simulink model "gm_Phase_voltages_per_switching_state_MPC_6Phase"  (R2022a)
settings: Solver=FixedStepDiscrete  StartTime=0.0  StopTime=10.0  RelTol=1e-3
undefined symbols (not defined in the file or in its folder): f_c, u_dc
libraries: hdlmdlgenlib x9
settings Model: Creator=Andre Merx  LastModifiedBy=Andre Merx
settings SolverCC: AlgebraicLoopSolver=TrustRegion
settings DataIOCC: LimitDataPoints=on  SaveOutput=off  SaveTime=off
settings OptimizationCC: BlockReduction=off  ConditionallyExecuteInputs=off  DefaultParameterBehavior=Inlined  LifeSpan=inf
settings DebuggingCC: AlgebraicLoopMsg=error  InheritedTsInSrcMsg=none  SingleTaskRateTransMsg=error  UnconnectedInputMsg=warning  UnconnectedOutputMsg=warning  UnconnectedLineMsg=warning  AllowSymbolicDim=off  StrictBusMsg=ErrorOnBusTreatedAsVector  SFUnexpectedBacktrackingDiag=warning  SFNoUnconditionalDefaultTransitionDiag=warning  SFExecutionAtInitializationDiag=none  SFMachineParentedDataDiag=warning  ArithmeticOperatorsInVariantConditions=warning
settings HardwareCC: ProdBitPerPointer=32  ProdBitPerSizeT=32  ProdBitPerPtrDiffT=32  ProdLargestAtomicFloat=None  ProdIntDivRoundTo=Undefined  ProdEndianess=Unspecified  ProdWordSize=32  ProdHWDeviceType=ASIC/FPGA->ASIC/FPGA  ProdEqTarget=off
settings SFSimCC: SimUseLocalCustomCode=off  CustomCodeUndefinedFunction=UseInterfaceOnly
settings RTWCC: RTWUseLocalCustomCode=off
settings CodeAppCC: StateflowObjectComments=on
settings GRTTargetCC: TargetLangStandard=C89/C90 (ANSI)
settings ConfigComp: CovScope=ReferencedModels  CovMetricSettings=dw  CovSaveCumulativeToWorkspaceVar=on  CovSaveSingleToWorkspaceVar=on  CovExternalEMLEnable=off  CovSFcnEnable=off

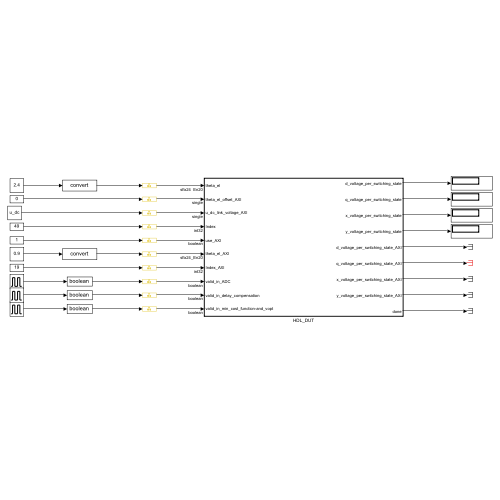
[thumbnail: Simulink's stored preview of the top-level diagram]
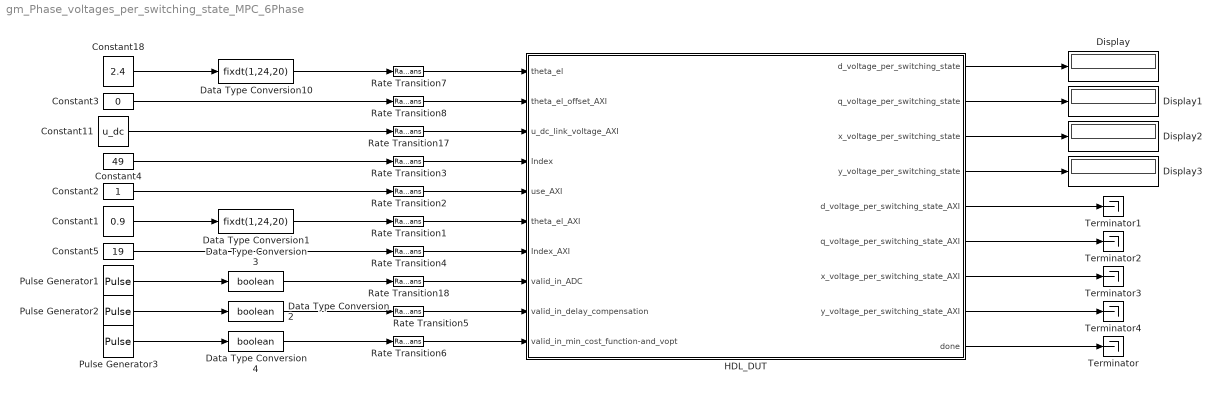
== system gm_Phase_voltages_per_switching_state_MPC_6Phase ==
  Constant1 : Constant  Value=0.9
  Constant11 : Constant  Value=u_dc  OutDataTypeStr=single  SampleTime=-1
  Constant18 : Constant  Value=2.4
  Constant2 : Constant  OutDataTypeStr=boolean  SampleTime=-1
  Constant3 : Constant  Value=0  OutDataTypeStr=single  SampleTime=-1
  Constant4 : Constant  Value=49  OutDataTypeStr=int32  SampleTime=-1
  Constant5 : Constant  Value=19  OutDataTypeStr=int32  SampleTime=-1
  Data Type Conversion1 : DataTypeConversion  OutDataTypeStr=fixdt(1,24,20)  SaturateOnIntegerOverflow=off  RndMeth=Floor
  Data Type Conversion10 : DataTypeConversion  OutDataTypeStr=fixdt(1,24,20)  SaturateOnIntegerOverflow=off  RndMeth=Floor
  Data Type Conversion2 : DataTypeConversion  OutDataTypeStr=boolean  SaturateOnIntegerOverflow=off  RndMeth=Floor
  Data Type Conversion3 : DataTypeConversion  OutDataTypeStr=boolean  SaturateOnIntegerOverflow=off  RndMeth=Floor
  Data Type Conversion4 : DataTypeConversion  OutDataTypeStr=boolean  SaturateOnIntegerOverflow=off  RndMeth=Floor
  Display{,1..3} (4 alike) : Display
  HDL_DUT : Subsystem  TreatAsAtomicUnit=on
  Pulse Generator1 : DiscretePulseGenerator  PulseType=Time based  Period=1/f_c
  Pulse Generator2 : DiscretePulseGenerator  PulseType=Time based  Period=1/f_c
  Pulse Generator3 : DiscretePulseGenerator  PulseType=Time based  Period=1/f_c
  Rate Transition{1..8,17..18} (10 alike) : RateTransition  OutPortSampleTime=Rt
  Terminator{,1..4} (5 alike) : Terminator
  wires:
  HDL_DUT/9(done) -> Terminator/1
  Rate Transition6/1 -> HDL_DUT/10(valid_in_min_cost_function-and_vopt)
  Data Type Conversion4/1 -> Rate Transition6/1
  Pulse Generator3/1 -> Data Type Conversion4/1
  Rate Transition5/1 -> HDL_DUT/9(valid_in_delay_compensation)
  Data Type Conversion2/1 -> Rate Transition5/1
  Pulse Generator2/1 -> Data Type Conversion2/1
  HDL_DUT/8(y_voltage_per_switching_state_AXI) -> Terminator4/1
  HDL_DUT/7(x_voltage_per_switching_state_AXI) -> Terminator3/1
  HDL_DUT/6(q_voltage_per_switching_state_AXI) -> Terminator2/1
  HDL_DUT/5(d_voltage_per_switching_state_AXI) -> Terminator1/1
  Rate Transition4/1 -> HDL_DUT/7(Index_AXI)
  Constant5/1 -> Rate Transition4/1
  Rate Transition3/1 -> HDL_DUT/4(Index)
  Constant4/1 -> Rate Transition3/1
  HDL_DUT/4(y_voltage_per_switching_state) -> Display3/1
  HDL_DUT/3(x_voltage_per_switching_state) -> Display2/1
  HDL_DUT/2(q_voltage_per_switching_state) -> Display1/1
  HDL_DUT/1(d_voltage_per_switching_state) -> Display/1
  Rate Transition2/1 -> HDL_DUT/5(use_AXI)
  Constant2/1 -> Rate Transition2/1
  Rate Transition1/1 -> HDL_DUT/6(theta_el_AXI)
  Constant1/1 -> Data Type Conversion1/1
  Data Type Conversion1/1 -> Rate Transition1/1
  Rate Transition18/1 -> HDL_DUT/8(valid_in_ADC)
  Data Type Conversion3/1 -> Rate Transition18/1
  Pulse Generator1/1 -> Data Type Conversion3/1
  Rate Transition8/1 -> HDL_DUT/2(theta_el_offset_AXI)
  Constant18/1 -> Data Type Conversion10/1
  Constant3/1 -> Rate Transition8/1
  Rate Transition7/1 -> HDL_DUT/1(theta_el)
  Rate Transition17/1 -> HDL_DUT/3(u_dc_link_voltage_AXI)
  Data Type Conversion10/1 -> Rate Transition7/1
  Constant11/1 -> Rate Transition17/1

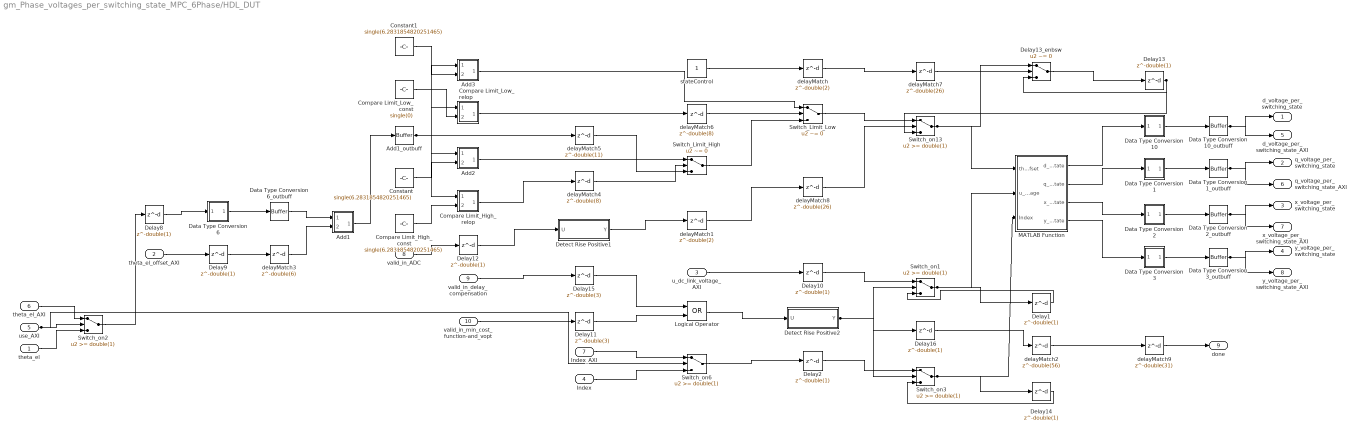
== system gm_Phase_voltages_per_switching_state_MPC_6Phase/HDL_DUT ==
  theta_el : Inport  OutDataTypeStr=fixdt(1, 24, 20)  PortDimensions=1  SampleTime=1e-08
  theta_el_offset_AXI : Inport  Port=2  OutDataTypeStr=single  PortDimensions=1  SampleTime=1e-08
  u_dc_link_voltage_AXI : Inport  Port=3  OutDataTypeStr=single  PortDimensions=1  SampleTime=1e-08
  Index : Inport  Port=4  OutDataTypeStr=int32  PortDimensions=1  SampleTime=1e-08
  use_AXI : Inport  Port=5  OutDataTypeStr=boolean  PortDimensions=1  SampleTime=1e-08
  theta_el_AXI : Inport  Port=6  OutDataTypeStr=fixdt(1, 24, 20)  PortDimensions=1  SampleTime=1e-08
  Index_AXI : Inport  Port=7  OutDataTypeStr=int32  PortDimensions=1  SampleTime=1e-08
  valid_in_ADC : Inport  Port=8  OutDataTypeStr=boolean  PortDimensions=1  SampleTime=1e-08
  valid_in_delay_compensation : Inport  Port=9  OutDataTypeStr=boolean  PortDimensions=1  SampleTime=1e-08
  valid_in_min_cost_function-and_vopt : Inport  Port=10  OutDataTypeStr=boolean  PortDimensions=1  SampleTime=1e-08
  Add1 : Subsystem
      mask Display: disp('NFP\nadd');
  Add1_outbuff : hdlmdlgenlib/Buffer
      settings: SourceProductBaseCode=SL
  Add2 : Subsystem
      mask Display: disp('NFP\nadd');
  Add3 : Subsystem
      mask Display: disp('NFP\nadd');
  Compare Limit_High_const : Constant  Value=single(6.2831854820251465)  OutDataTypeStr=single  SampleTime=1e-08
  Compare Limit_High_relop : Subsystem
      mask Display: disp('NFP\nrelop');
  Compare Limit_Low_const : Constant  Value=single(0)  OutDataTypeStr=single  SampleTime=1e-08
  Compare Limit_Low_relop : Subsystem
      mask Display: disp('NFP\nrelop');
  Constant : Constant  Value=single(6.2831854820251465)  OutDataTypeStr=single  SampleTime=1e-08
  Constant1 : Constant  Value=single(6.2831854820251465)  OutDataTypeStr=single  SampleTime=1e-08
  Data Type Conversion1 : Subsystem
      mask Display: disp('NFP\nconv');
  Data Type Conversion10 : Subsystem
      mask Display: disp('NFP\nconv');
  Data Type Conversion10_outbuff : hdlmdlgenlib/Buffer
      settings: SourceProductBaseCode=SL
  Data Type Conversion1_outbuff : hdlmdlgenlib/Buffer
      settings: SourceProductBaseCode=SL
  Data Type Conversion2 : Subsystem
      mask Display: disp('NFP\nconv');
  Data Type Conversion2_outbuff : hdlmdlgenlib/Buffer
      settings: SourceProductBaseCode=SL
  Data Type Conversion3 : Subsystem
      mask Display: disp('NFP\nconv');
  Data Type Conversion3_outbuff : hdlmdlgenlib/Buffer
      settings: SourceProductBaseCode=SL
  Data Type Conversion6 : Subsystem
      mask Display: disp('NFP\nconv');
  Data Type Conversion6_outbuff : hdlmdlgenlib/Buffer
      settings: SourceProductBaseCode=SL
  Delay{1..2,8..10,12..14,16} (9 alike) : Delay  DelayLength=double(1)  InitialCondition=0  SampleTime=1e-08
  Delay11 : Delay  DelayLength=double(3)  InitialCondition=0  SampleTime=1e-08
  Delay13_enbsw : Switch  Criteria=u2 ~= 0  Threshold=double(0)  OutDataTypeStr=single  SampleTime=1e-08  SaturateOnIntegerOverflow=off  InputSameDT=off
  Delay15 : Delay  DelayLength=double(3)  InitialCondition=0  SampleTime=1e-08
  Detect Rise Positive1 : Subsystem  mask(Detect Rise Positive){vinit=double(0), InputProcessing=Elements as channels (sample based), OutDataTypeStr=boolean}
      mask prompts: vinit "Simulink:masks:InitialCondition_MP"; InputProcessing "Simulink:masks:InputProcessing_MP"; OutDataTypeStr "Simulink:masks:OutputDataType_MP"
      mask help: Simulink:masks:DetectRisePositive_MD
      mask init:
      | InputProcessing = 'Elements as channels (sample based)';
      | OutDataTypeStr = 'boolean';
      | vinit = double(0);
      mask TypeOptions InputProcessing: Simulink:masks:ColumnsAsChannelsFrameBased | Simulink:masks:ElementsAsChannelsSampleBased
      mask TypeOptions OutDataTypeStr: Simulink:masks:uint8 | Simulink:masks:boolean
      mask Display: fprintf('U > 0\n&  NOT\nU/z > 0')
  Detect Rise Positive2 : Subsystem  mask(Detect Rise Positive){vinit=double(0), InputProcessing=Elements as channels (sample based), OutDataTypeStr=boolean}
      mask prompts: vinit "Simulink:masks:InitialCondition_MP"; InputProcessing "Simulink:masks:InputProcessing_MP"; OutDataTypeStr "Simulink:masks:OutputDataType_MP"
      mask help: Simulink:masks:DetectRisePositive_MD
      mask init:
      | InputProcessing = 'Elements as channels (sample based)';
      | OutDataTypeStr = 'boolean';
      | vinit = double(0);
      mask TypeOptions InputProcessing: Simulink:masks:ColumnsAsChannelsFrameBased | Simulink:masks:ElementsAsChannelsSampleBased
      mask TypeOptions OutDataTypeStr: Simulink:masks:uint8 | Simulink:masks:boolean
      mask Display: fprintf('U > 0\n&  NOT\nU/z > 0')
  Logical Operator : Logic  Operator=OR  AllPortsSameDT=off  OutDataTypeStr=boolean  SampleTime=1e-08
  MATLAB Function : Subsystem
  Switch_Limit_High : Switch  Criteria=u2 ~= 0  Threshold=double(0)  OutDataTypeStr=single  SampleTime=1e-08  SaturateOnIntegerOverflow=off  InputSameDT=off
  Switch_Limit_Low : Switch  Criteria=u2 ~= 0  Threshold=double(0)  OutDataTypeStr=single  SampleTime=1e-08  SaturateOnIntegerOverflow=off  InputSameDT=off
  Switch_on1 : Switch  Threshold=double(1)  OutDataTypeStr=single  RndMeth=Simplest  SampleTime=1e-08  SaturateOnIntegerOverflow=off  InputSameDT=off
  Switch_on13 : Switch  Threshold=double(1)  OutDataTypeStr=single  RndMeth=Simplest  SampleTime=1e-08  SaturateOnIntegerOverflow=off  InputSameDT=off
  Switch_on2 : Switch  Threshold=double(1)  OutDataTypeStr=fixdt(1, 24, 20)  RndMeth=Simplest  SampleTime=1e-08  SaturateOnIntegerOverflow=off  InputSameDT=off
  Switch_on3 : Switch  Threshold=double(1)  OutDataTypeStr=int32  RndMeth=Simplest  SampleTime=1e-08  SaturateOnIntegerOverflow=off  InputSameDT=off
  Switch_on6 : Switch  Threshold=double(1)  OutDataTypeStr=int32  RndMeth=Simplest  SampleTime=1e-08  SaturateOnIntegerOverflow=off  InputSameDT=off
  delayMatch : Delay  DelayLength=double(2)  InitialCondition=0  SampleTime=1e-08
  delayMatch1 : Delay  DelayLength=double(2)  InitialCondition=0  SampleTime=1e-08
  delayMatch2 : Delay  DelayLength=double(56)  InitialCondition=0  SampleTime=1e-08
  delayMatch3 : Delay  DelayLength=double(6)  InitialCondition=0  SampleTime=1e-08
  delayMatch4 : Delay  DelayLength=double(8)  InitialCondition=0  SampleTime=1e-08
  delayMatch5 : Delay  DelayLength=double(11)  InitialCondition=0  SampleTime=1e-08
  delayMatch6 : Delay  DelayLength=double(8)  InitialCondition=0  SampleTime=1e-08
  delayMatch7 : Delay  DelayLength=double(26)  InitialCondition=0  SampleTime=1e-08
  delayMatch8 : Delay  DelayLength=double(26)  InitialCondition=0  SampleTime=1e-08
  delayMatch9 : Delay  DelayLength=double(31)  InitialCondition=0  SampleTime=1e-08
  stateControl : Constant  OutDataTypeStr=boolean  SampleTime=1e-08
  d_voltage_per_switching_state : Outport  SampleTime=1e-08
  q_voltage_per_switching_state : Outport  Port=2  SampleTime=1e-08
  x_voltage_per_switching_state : Outport  Port=3  SampleTime=1e-08
  y_voltage_per_switching_state : Outport  Port=4  SampleTime=1e-08
  d_voltage_per_switching_state_AXI : Outport  Port=5  SampleTime=1e-08
  q_voltage_per_switching_state_AXI : Outport  Port=6  SampleTime=1e-08
  x_voltage_per_switching_state_AXI : Outport  Port=7  SampleTime=1e-08
  y_voltage_per_switching_state_AXI : Outport  Port=8  SampleTime=1e-08
  done : Outport  Port=9  SampleTime=1e-08
  wires:
  theta_el/1 -> Switch_on2/3
  theta_el_offset_AXI/1 -> Delay9/1
  u_dc_link_voltage_AXI/1 -> Delay10/1
  Index/1 -> Switch_on6/3
  use_AXI/1 -> Switch_on6/2, Switch_on2/2
  theta_el_AXI/1 -> Switch_on2/1
  Index_AXI/1 -> Switch_on6/1
  valid_in_ADC/1 -> Delay12/1
  valid_in_delay_compensation/1 -> Delay15/1
  valid_in_min_cost_function-and_vopt/1 -> Delay11/1
  delayMatch5/1 -> Switch_Limit_High/3
  Constant/1 -> Add2/2(In2)
  Constant1/1 -> Add3/2(In2)
  Data Type Conversion1_outbuff/1 -> q_voltage_per_switching_state/1, q_voltage_per_switching_state_AXI/1
  Data Type Conversion10_outbuff/1 -> d_voltage_per_switching_state_AXI/1, d_voltage_per_switching_state/1
  Data Type Conversion2_outbuff/1 -> x_voltage_per_switching_state_AXI/1, x_voltage_per_switching_state/1
  Data Type Conversion3_outbuff/1 -> y_voltage_per_switching_state/1, y_voltage_per_switching_state_AXI/1
  Data Type Conversion6_outbuff/1 -> Add1/1(In1)
  Delay10/1 -> Switch_on1/1
  Delay11/1 -> Logical Operator/2
  Delay12/1 -> Detect Rise Positive1/1(U)
  Delay15/1 -> Logical Operator/1
  delayMatch9/1 -> done/1
  Delay2/1 -> Switch_on3/1
  Delay8/1 -> Data Type Conversion6/1(In1)
  delayMatch3/1 -> Add1/2(In2)
  delayMatch8/1 -> Switch_on13/2
  Detect Rise Positive2/1(Y) -> Delay16/1, Switch_on1/2, Switch_on3/2
  Logical Operator/1 -> Detect Rise Positive2/1(U)
  MATLAB Function/1(d_voltage_per_switching_state) -> Data Type Conversion10/1(In1)
  MATLAB Function/2(q_voltage_per_switching_state) -> Data Type Conversion1/1(In1)
  MATLAB Function/3(x_voltage_per_switching_state) -> Data Type Conversion2/1(In1)
  MATLAB Function/4(y_voltage_per_switching_state) -> Data Type Conversion3/1(In1)
  Switch_Limit_High/1 -> Switch_Limit_Low/3
  Switch_Limit_Low/1 -> Switch_on13/1
  Switch_on1/1 -> MATLAB Function/2(u_dc_link_voltage), Delay1/1
  Switch_on2/1 -> Delay8/1
  Switch_on3/1 -> MATLAB Function/3(Index), Delay14/1
  Switch_on6/1 -> Delay2/1
  Add1_outbuff/1 -> Compare Limit_Low_relop/1(In1), Compare Limit_High_relop/1(In1), Add3/1(In1), Add2/1(In1), delayMatch5/1
  delayMatch4/1 -> Switch_Limit_High/2
  delayMatch6/1 -> Switch_Limit_Low/2
  Compare Limit_High_const/1 -> Compare Limit_High_relop/2(In2)
  Compare Limit_Low_const/1 -> Compare Limit_Low_relop/2(In2)
  delayMatch7/1 -> Delay13_enbsw/2
  stateControl/1 -> delayMatch/1
  Detect Rise Positive1/1(Y) -> delayMatch1/1
  Delay16/1 -> delayMatch2/1
  Add1/1(Out1) -> Add1_outbuff/1
  Add2/1(Out1) -> Switch_Limit_High/1
  Add3/1(Out1) -> Switch_Limit_Low/1
  Compare Limit_High_relop/1(Out1) -> delayMatch4/1
  Compare Limit_Low_relop/1(Out1) -> delayMatch6/1
  Data Type Conversion1/1(Out1) -> Data Type Conversion1_outbuff/1
  Data Type Conversion10/1(Out1) -> Data Type Conversion10_outbuff/1
  Data Type Conversion2/1(Out1) -> Data Type Conversion2_outbuff/1
  Data Type Conversion3/1(Out1) -> Data Type Conversion3_outbuff/1
  Data Type Conversion6/1(Out1) -> Data Type Conversion6_outbuff/1
  Delay9/1 -> delayMatch3/1
  delayMatch/1 -> delayMatch7/1
  delayMatch1/1 -> delayMatch8/1
  delayMatch2/1 -> delayMatch9/1
  Switch_on13/1 -> MATLAB Function/1(theta_el_with_offset), Delay13_enbsw/1
  Delay13_enbsw/1 -> Delay13/1
  Delay13/1 -> Switch_on13/3, Delay13_enbsw/3
  Delay1/1 -> Switch_on1/3
  Delay14/1 -> Switch_on3/3

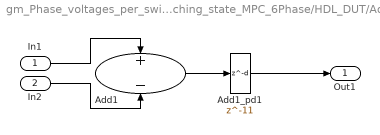
== system gm_Phase_voltages_per_switching_state_MPC_6Phase/HDL_DUT/Add1 ==
  In1 : Inport
  In2 : Inport  Port=2
  Add1 : Sum  Inputs=+-  OutDataTypeStr=single  SampleTime=1e-08
  Add1_pd1 : Delay  DelayLength=11
  Out1 : Outport
  wires:
  In1/1 -> Add1/1
  In2/1 -> Add1/2
  Add1/1 -> Add1_pd1/1
  Add1_pd1/1 -> Out1/1

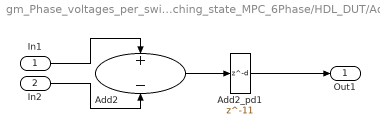
== system gm_Phase_voltages_per_switching_state_MPC_6Phase/HDL_DUT/Add2 ==
  In1 : Inport
  In2 : Inport  Port=2
  Add2 : Sum  Inputs=+-  OutDataTypeStr=single  SampleTime=1e-08
  Add2_pd1 : Delay  DelayLength=11
  Out1 : Outport
  wires:
  In1/1 -> Add2/1
  In2/1 -> Add2/2
  Add2/1 -> Add2_pd1/1
  Add2_pd1/1 -> Out1/1

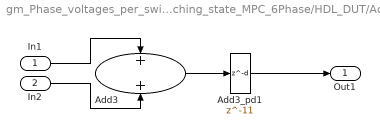
== system gm_Phase_voltages_per_switching_state_MPC_6Phase/HDL_DUT/Add3 ==
  In1 : Inport
  In2 : Inport  Port=2
  Add3 : Sum  OutDataTypeStr=single  SampleTime=1e-08
  Add3_pd1 : Delay  DelayLength=11
  Out1 : Outport
  wires:
  In1/1 -> Add3/1
  In2/1 -> Add3/2
  Add3/1 -> Add3_pd1/1
  Add3_pd1/1 -> Out1/1

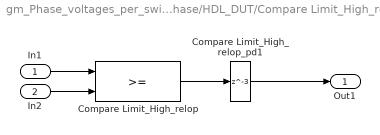
== system gm_Phase_voltages_per_switching_state_MPC_6Phase/HDL_DUT/Compare Limit_High_relop ==
  In1 : Inport
  In2 : Inport  Port=2
  Compare Limit_High_relop : RelationalOperator  OutDataTypeStr=boolean  SampleTime=1e-08
  Compare Limit_High_relop_pd1 : Delay  DelayLength=3
  Out1 : Outport
  wires:
  In1/1 -> Compare Limit_High_relop/1
  In2/1 -> Compare Limit_High_relop/2
  Compare Limit_High_relop/1 -> Compare Limit_High_relop_pd1/1
  Compare Limit_High_relop_pd1/1 -> Out1/1

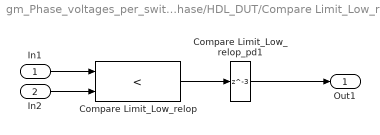
== system gm_Phase_voltages_per_switching_state_MPC_6Phase/HDL_DUT/Compare Limit_Low_relop ==
  In1 : Inport
  In2 : Inport  Port=2
  Compare Limit_Low_relop : RelationalOperator  Operator=<  OutDataTypeStr=boolean  SampleTime=1e-08
  Compare Limit_Low_relop_pd1 : Delay  DelayLength=3
  Out1 : Outport
  wires:
  In1/1 -> Compare Limit_Low_relop/1
  In2/1 -> Compare Limit_Low_relop/2
  Compare Limit_Low_relop/1 -> Compare Limit_Low_relop_pd1/1
  Compare Limit_Low_relop_pd1/1 -> Out1/1

== system gm_Phase_voltages_per_switching_state_MPC_6Phase/HDL_DUT/Data Type Conversion1 ==
  In1 : Inport
  Data Type Conversion1 : DataTypeConversion  OutDataTypeStr=fixdt(1, 24, 11)  SampleTime=1e-08  SaturateOnIntegerOverflow=off  RndMeth=Floor
  Data Type Conversion1_pd1 : Delay  DelayLength=6
  Out1 : Outport
  wires:
  In1/1 -> Data Type Conversion1/1
  Data Type Conversion1/1 -> Data Type Conversion1_pd1/1
  Data Type Conversion1_pd1/1 -> Out1/1

== system gm_Phase_voltages_per_switching_state_MPC_6Phase/HDL_DUT/Data Type Conversion10 ==
  In1 : Inport
  Data Type Conversion10 : DataTypeConversion  OutDataTypeStr=fixdt(1, 24, 11)  SampleTime=1e-08  SaturateOnIntegerOverflow=off  RndMeth=Floor
  Data Type Conversion10_pd1 : Delay  DelayLength=6
  Out1 : Outport
  wires:
  In1/1 -> Data Type Conversion10/1
  Data Type Conversion10/1 -> Data Type Conversion10_pd1/1
  Data Type Conversion10_pd1/1 -> Out1/1

== system gm_Phase_voltages_per_switching_state_MPC_6Phase/HDL_DUT/Data Type Conversion2 ==
  In1 : Inport
  Data Type Conversion2 : DataTypeConversion  OutDataTypeStr=fixdt(1, 24, 11)  SampleTime=1e-08  SaturateOnIntegerOverflow=off  RndMeth=Floor
  Data Type Conversion2_pd1 : Delay  DelayLength=6
  Out1 : Outport
  wires:
  In1/1 -> Data Type Conversion2/1
  Data Type Conversion2/1 -> Data Type Conversion2_pd1/1
  Data Type Conversion2_pd1/1 -> Out1/1

== system gm_Phase_voltages_per_switching_state_MPC_6Phase/HDL_DUT/Data Type Conversion3 ==
  In1 : Inport
  Data Type Conversion3 : DataTypeConversion  OutDataTypeStr=fixdt(1, 24, 11)  SampleTime=1e-08  SaturateOnIntegerOverflow=off  RndMeth=Floor
  Data Type Conversion3_pd1 : Delay  DelayLength=6
  Out1 : Outport
  wires:
  In1/1 -> Data Type Conversion3/1
  Data Type Conversion3/1 -> Data Type Conversion3_pd1/1
  Data Type Conversion3_pd1/1 -> Out1/1

== system gm_Phase_voltages_per_switching_state_MPC_6Phase/HDL_DUT/Data Type Conversion6 ==
  In1 : Inport
  Data Type Conversion6 : DataTypeConversion  OutDataTypeStr=single  RndMeth=Nearest  SampleTime=1e-08  SaturateOnIntegerOverflow=off
  Data Type Conversion6_pd1 : Delay  DelayLength=6
  Out1 : Outport
  wires:
  In1/1 -> Data Type Conversion6/1
  Data Type Conversion6/1 -> Data Type Conversion6_pd1/1
  Data Type Conversion6_pd1/1 -> Out1/1

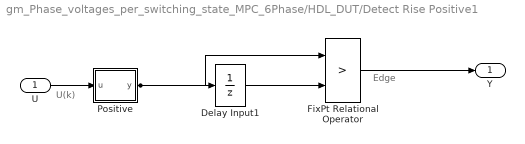
== system gm_Phase_voltages_per_switching_state_MPC_6Phase/HDL_DUT/Detect Rise Positive1 ==
  note: Edge
  note: U(k)
  U : Inport  OutDataTypeStr=boolean  SampleTime=1e-08
  Delay Input1 : UnitDelay  Description=Store in Global RAM  DisableCoverage=on  InitialCondition=vinit  SampleTime=-1  HasFrameUpgradeWarning=on
  FixPt Relational Operator : RelationalOperator  Operator=>  OutDataTypeStr=boolean  ZeroCross=off  InputSameDT=off
  Positive : Subsystem  mask(Compare To Zero){relop=>, OutDataTypeStr=boolean, ZeroCross=off}
      mask prompts: relop "Simulink:masks:Operator_MP"; OutDataTypeStr "Simulink:masks:OutputDataType_MP"; ZeroCross "Simulink:masks:EnableZerocrossingDetection_MP"
      mask help: Simulink:masks:CompareToZero_MD
      mask init:
      | OutDataTypeStr = 'boolean';
      | ZeroCross = 'off';
      | blkName = 'Phase_voltages_per_switching_state_MPC_6Phase/HDL_DUT/Detect Rise\nPositive1/Positive';
      | relop = '>';
      | setValue = 'boolean';
      mask TypeOptions relop: == | ~= | < | <= | >= | >
      mask TypeOptions OutDataTypeStr: Simulink:masks:uint8 | Simulink:masks:boolean
      mask Callback ZeroCross: sl('zeroCrossEnable', gcbh);
      mask Display: disp([relop,' 0'])
  Y : Outport  SampleTime=1e-08
  wires:
  Delay Input1/1 -> FixPt Relational Operator/2
  FixPt Relational Operator/1 -> Y/1
  Positive/1(y) -> FixPt Relational Operator/1, Delay Input1/1
  U/1 -> Positive/1(u)

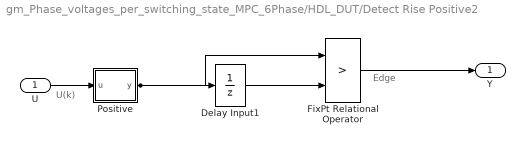
== system gm_Phase_voltages_per_switching_state_MPC_6Phase/HDL_DUT/Detect Rise Positive2 ==
  note: Edge
  note: U(k)
  U : Inport  OutDataTypeStr=boolean  SampleTime=1e-08
  Delay Input1 : UnitDelay  Description=Store in Global RAM  DisableCoverage=on  InitialCondition=vinit  SampleTime=-1  HasFrameUpgradeWarning=on
  FixPt Relational Operator : RelationalOperator  Operator=>  OutDataTypeStr=boolean  ZeroCross=off  InputSameDT=off
  Positive : Subsystem  mask(Compare To Zero){relop=>, OutDataTypeStr=boolean, ZeroCross=off}
      mask prompts: relop "Simulink:masks:Operator_MP"; OutDataTypeStr "Simulink:masks:OutputDataType_MP"; ZeroCross "Simulink:masks:EnableZerocrossingDetection_MP"
      mask help: Simulink:masks:CompareToZero_MD
      mask init:
      | OutDataTypeStr = 'boolean';
      | ZeroCross = 'off';
      | blkName = 'Phase_voltages_per_switching_state_MPC_6Phase/HDL_DUT/Detect Rise\nPositive2/Positive';
      | relop = '>';
      | setValue = 'boolean';
      mask TypeOptions relop: == | ~= | < | <= | >= | >
      mask TypeOptions OutDataTypeStr: Simulink:masks:uint8 | Simulink:masks:boolean
      mask Callback ZeroCross: sl('zeroCrossEnable', gcbh);
      mask Display: disp([relop,' 0'])
  Y : Outport  SampleTime=1e-08
  wires:
  Delay Input1/1 -> FixPt Relational Operator/2
  FixPt Relational Operator/1 -> Y/1
  Positive/1(y) -> FixPt Relational Operator/1, Delay Input1/1
  U/1 -> Positive/1(u)

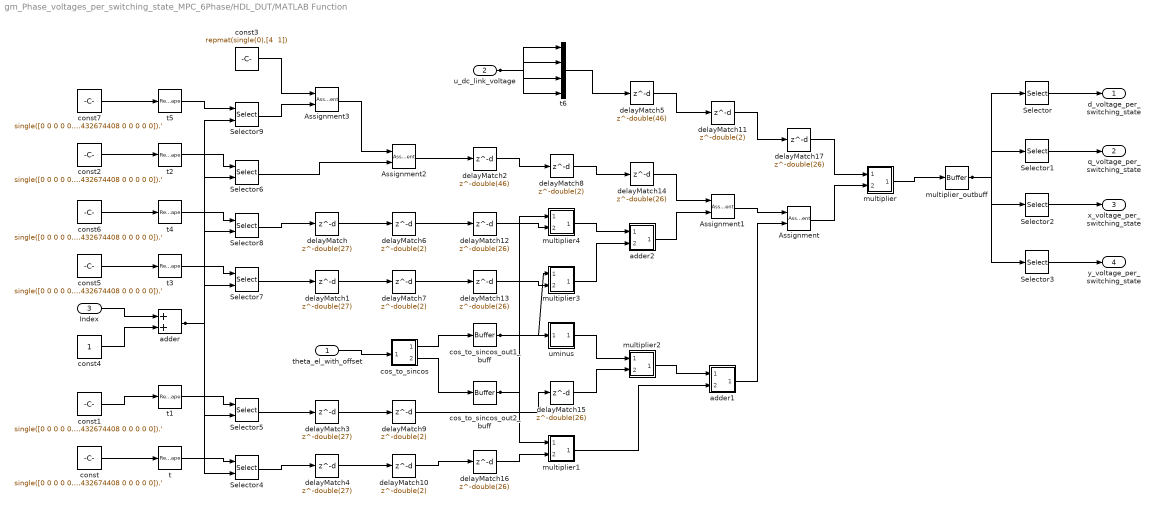
== system gm_Phase_voltages_per_switching_state_MPC_6Phase/HDL_DUT/MATLAB Function ==
  theta_el_with_offset : Inport  OutDataTypeStr=single  PortDimensions=1  SampleTime=1e-08
  u_dc_link_voltage : Inport  Port=2  OutDataTypeStr=single  PortDimensions=1  SampleTime=1e-08
  Index : Inport  Port=3  OutDataTypeStr=int32  PortDimensions=1  SampleTime=1e-08
  Assignment : Assignment  NumberOfDimensions=2  SampleTime=1e-08  IndexOptions=Index vector (dialog),Index vector (dialog)  Indices=double(2),double(1)  OutputSizes=double(0),double(0)
  Assignment1 : Assignment  NumberOfDimensions=2  SampleTime=1e-08  IndexOptions=Index vector (dialog),Index vector (dialog)  Indices=double(1),double(1)  OutputSizes=double(0),double(0)
  Assignment2 : Assignment  NumberOfDimensions=2  SampleTime=1e-08  IndexOptions=Index vector (dialog),Index vector (dialog)  Indices=double(4),double(1)  OutputSizes=double(0),double(0)
  Assignment3 : Assignment  NumberOfDimensions=2  SampleTime=1e-08  IndexOptions=Index vector (dialog),Index vector (dialog)  Indices=double(3),double(1)  OutputSizes=double(0),double(0)
  Selector : Selector  NumberOfDimensions=2  SampleTime=1e-08  IndexOptions=Index vector (dialog),Index vector (dialog)  Indices=double(1),double(1)  OutputSizes=double(0),double(0)
  Selector1 : Selector  NumberOfDimensions=2  SampleTime=1e-08  IndexOptions=Index vector (dialog),Index vector (dialog)  Indices=double(2),double(1)  OutputSizes=double(0),double(0)
  Selector2 : Selector  NumberOfDimensions=2  SampleTime=1e-08  IndexOptions=Index vector (dialog),Index vector (dialog)  Indices=double(3),double(1)  OutputSizes=double(0),double(0)
  Selector3 : Selector  NumberOfDimensions=2  SampleTime=1e-08  IndexOptions=Index vector (dialog),Index vector (dialog)  Indices=double(4),double(1)  OutputSizes=double(0),double(0)
  Selector4 : Selector  NumberOfDimensions=2  SampleTime=1e-08  IndexOptions=Index vector (dialog),Index vector (port)  Indices=double(2),double(-1)  OutputSizes=double(0),double(0)
  Selector5 : Selector  NumberOfDimensions=2  SampleTime=1e-08  IndexOptions=Index vector (dialog),Index vector (port)  Indices=double(1),double(-1)  OutputSizes=double(0),double(0)
  Selector6 : Selector  NumberOfDimensions=2  SampleTime=1e-08  IndexOptions=Index vector (dialog),Index vector (port)  Indices=double(4),double(-1)  OutputSizes=double(0),double(0)
  Selector7 : Selector  NumberOfDimensions=2  SampleTime=1e-08  IndexOptions=Index vector (dialog),Index vector (port)  Indices=double(2),double(-1)  OutputSizes=double(0),double(0)
  Selector8 : Selector  NumberOfDimensions=2  SampleTime=1e-08  IndexOptions=Index vector (dialog),Index vector (port)  Indices=double(1),double(-1)  OutputSizes=double(0),double(0)
  Selector9 : Selector  NumberOfDimensions=2  SampleTime=1e-08  IndexOptions=Index vector (dialog),Index vector (port)  Indices=double(3),double(-1)  OutputSizes=double(0),double(0)
  adder : Sum  AccumDataTypeStr=int32  OutDataTypeStr=int32  RndMeth=Nearest  SaturateOnIntegerOverflow=on  SampleTime=1e-08
  adder1 : Subsystem
      mask Display: disp('NFP\nadd');
  adder2 : Subsystem
      mask Display: disp('NFP\nadd');
  const{,1..2,5..7} (6 alike) : Constant  Value=single([0 0 0 0 0.3333333432674408 0 0.3333333432674408 0 -0.1666666716337204 0.28867512941360474 -0.1666666716337204 -0.28867512941360474 0.1666666716337204 0.28867512941360474 0.1666666716337204 -0.28867512941360474 -0.1666666716337204 -0.28867512941360474 -0.1666666716337204 0.28867512941360474 0.1666666716337204 -0.28867512941360474 0.1666666716337204 0.28867512941360474 -0.3333333432674408 0 -0.3333333432674408 0 0 0 0 0 0.28867512941360474 0.1666666716337204 -0.28867512941360474 0.1666666716337204 0.6220084428787231 0.1666666716337204 0.044658198952674866 0.1666666716337204 0.12200846523046494 0.45534181594848633 -0.45534181594848633 -0.12200846523046494 0.45534181594848633 0.45534181594848633 -0.12200846523046494 -0.12200846523046494 0.12200846523046494 -0.12200846523046494 -0.45534181594848633 0.45534181594848633 0.45534181594848633 -0.12200846523046494 -0.12200846523046494 0.45534181594848633 -0.044658198952674866 0.1666666716337204 -0.6220084428787231 0.1666666716337204 0.28867512941360474 0.1666666716337204 -0.28867512941360474 0.1666666716337204 -0.28867512941360474 0.1666666716337204 0.28867512941360474 0.1666666716337204 0.044658198952674866 0.1666666716337204 0.6220084428787231 0.1666666716337204 -0.45534181594848633 0.45534181594848633 0.12200846523046494 -0.12200846523046494 -0.12200846523046494 0.45534181594848633 0.45534181594848633 -0.12200846523046494 -0.45534181594848633 -0.12200846523046494 0.12200846523046494 0.45534181594848633 -0.12200846523046494 -0.12200846523046494 0.45534181594848633 0.45534181594848633 -0.6220084428787231 0.1666666716337204 -0.044658198952674866 0.1666666716337204 -0.28867512941360474 0.1666666716337204 0.28867512941360474 0.1666666716337204 0 0.3333333432674408 0 0.3333333432674408 0.3333333432674408 0.3333333432674408 0.3333333432674408 0.3333333432674408 -0.1666666716337204 0.6220084428787231 -0.1666666716337204 0.044658198952674866 0.1666666716337204 0.6220084428787231 0.1666666716337204 0.044658198952674866 -0.1666666716337204 0.044658198952674866 -0.1666666716337204 0.6220084428787231 0.1666666716337204 0.044658198952674866 0.1666666716337204 0.6220084428787231 -0.3333333432674408 0.3333333432674408 -0.3333333432674408 0.3333333432674408 0 0.3333333432674408 0 0.3333333432674408 0 -0.3333333432674408 0 -0.3333333432674408 0.3333333432674408 -0.3333333432674408 0.3333333432674408 -0.3333333432674408 -0.1666666716337204 -0.044658198952674866 -0.1666666716337204 -0.6220084428787231 0.1666666716337204 -0.044658198952674866 0.1666666716337204 -0.6220084428787231 -0.1666666716337204 -0.6220084428787231 -0.1666666716337204 -0.044658198952674866 0.1666666716337204 -0.6220084428787231 0.1666666716337204 -0.044658198952674866 -0.3333333432674408 -0.3333333432674408 -0.3333333432674408 -0.3333333432674408 0 -0.3333333432674408 0 -0.3333333432674408 0.28867512941360474 -0.1666666716337204 -0.28867512941360474 -0.1666666716337204 0.6220084428787231 -0.1666666716337204 0.044658198952674866 -0.1666666716337204 0.12200846523046494 0.12200846523046494 -0.45534181594848633 -0.45534181594848633 0.45534181594848633 0.12200846523046494 -0.12200846523046494 -0.45534181594848633 0.12200846523046494 -0.45534181594848633 -0.45534181594848633 0.12200846523046494 0.45534181594848633 -0.45534181594848633 -0.12200846523046494 0.12200846523046494 -0.044658198952674866 -0.1666666716337204 -0.6220084428787231 -0.1666666716337204 0.28867512941360474 -0.1666666716337204 -0.28867512941360474 -0.1666666716337204 -0.28867512941360474 -0.1666666716337204 0.28867512941360474 -0.1666666716337204 0.044658198952674866 -0.1666666716337204 0.6220084428787231 -0.1666666716337204 -0.45534181594848633 0.12200846523046494 0.12200846523046494 -0.45534181594848633 -0.12200846523046494 0.12200846523046494 0.45534181594848633 -0.45534181594848633 -0.45534181594848633 -0.45534181594848633 0.12200846523046494 0.12200846523046494 -0.12200846523046494 -0.45534181594848633 0.45534181594848633 0.12200846523046494 -0.6220084428787231 ...(+565 chars)]).'  VectorParams1D=off  OutDataTypeStr=single  SampleTime=1e-08
  const3 : Constant  Value="repmat(single(0),[4  1])"  VectorParams1D=off  OutDataTypeStr=single  SampleTime=1e-08
  const4 : Constant  VectorParams1D=off  OutDataTypeStr=int32  SampleTime=1e-08
  cos_to_sincos : Subsystem
      mask Display: disp('NFP\ntrig2');
  cos_to_sincos_out1_buff : hdlmdlgenlib/Buffer
      settings: SourceProductBaseCode=SL
  cos_to_sincos_out2_buff : hdlmdlgenlib/Buffer
      settings: SourceProductBaseCode=SL
  delayMatch{,1,3..4} (4 alike) : Delay  DelayLength=double(27)  InitialCondition=0  SampleTime=1e-08
  delayMatch{6..11} (6 alike) : Delay  DelayLength=double(2)  InitialCondition=0  SampleTime=1e-08
  delayMatch{12..17} (6 alike) : Delay  DelayLength=double(26)  InitialCondition=0  SampleTime=1e-08
  delayMatch2 : Delay  DelayLength=double(46)  InitialCondition=0  SampleTime=1e-08
  delayMatch5 : Delay  DelayLength=double(46)  InitialCondition=0  SampleTime=1e-08
  multiplier : Subsystem
      mask Display: disp('NFP\nmul');
  multiplier1 : Subsystem
      mask Display: disp('NFP\nmul');
  multiplier2 : Subsystem
      mask Display: disp('NFP\nmul');
  multiplier3 : Subsystem
      mask Display: disp('NFP\nmul');
  multiplier4 : Subsystem
      mask Display: disp('NFP\nmul');
  multiplier_outbuff : hdlmdlgenlib/Buffer
      settings: SourceProductBaseCode=SL
  t{,1..5} (6 alike) : Reshape  OutputDimensionality=Customize  OutputDimensions=[4,64]
  t6 : Mux
  uminus : Subsystem
      mask Display: disp('NFP\numinus');
  d_voltage_per_switching_state : Outport  SampleTime=1e-08  VectorParamsAs1DForOutWhenUnconnected=off
  q_voltage_per_switching_state : Outport  Port=2  SampleTime=1e-08
  x_voltage_per_switching_state : Outport  Port=3  SampleTime=1e-08
  y_voltage_per_switching_state : Outport  Port=4  SampleTime=1e-08
  wires:
  Selector/1 -> d_voltage_per_switching_state/1
  Selector1/1 -> q_voltage_per_switching_state/1
  Selector2/1 -> x_voltage_per_switching_state/1
  Selector3/1 -> y_voltage_per_switching_state/1
  multiplier_outbuff/1 -> Selector3/1, Selector2/1, Selector1/1, Selector/1
  Assignment/1 -> multiplier/2(In2)
  Assignment1/1 -> Assignment/1
  delayMatch14/1 -> Assignment1/1
  delayMatch16/1 -> multiplier1/2(In2)
  cos_to_sincos_out2_buff/1 -> multiplier4/1(In1), multiplier1/1(In1)
  delayMatch15/1 -> multiplier2/2(In2)
  Selector6/1 -> Assignment2/2
  Assignment3/1 -> Assignment2/1
  adder/1 -> Selector9/2, Selector8/2, Selector7/2, Selector6/2, Selector5/2, Selector4/2
  t/1 -> Selector4/1
  t1/1 -> Selector5/1
  cos_to_sincos_out1_buff/1 -> multiplier3/1(In1), uminus/1(In1)
  delayMatch13/1 -> multiplier3/2(In2)
  delayMatch12/1 -> multiplier4/2(In2)
  t2/1 -> Selector6/1
  Selector9/1 -> Assignment3/2
  const3/1 -> Assignment3/1
  const4/1 -> adder/2
  t3/1 -> Selector7/1
  t4/1 -> Selector8/1
  t5/1 -> Selector9/1
  const/1 -> t/1
  const1/1 -> t1/1
  const2/1 -> t2/1
  const5/1 -> t3/1
  const6/1 -> t4/1
  const7/1 -> t5/1
  delayMatch17/1 -> multiplier/1(In1)
  multiplier/1(Out1) -> multiplier_outbuff/1
  adder1/1(Out1) -> Assignment/2
  multiplier1/1(Out1) -> adder1/2(In2)
  multiplier2/1(Out1) -> adder1/1(In1)
  adder2/1(Out1) -> Assignment1/2
  uminus/1(Out1) -> multiplier2/1(In1)
  multiplier3/1(Out1) -> adder2/2(In2)
  multiplier4/1(Out1) -> adder2/1(In1)
  cos_to_sincos/1(Out1) -> cos_to_sincos_out1_buff/1
  cos_to_sincos/2(Out2) -> cos_to_sincos_out2_buff/1
  Selector8/1 -> delayMatch/1
  Selector7/1 -> delayMatch1/1
  Assignment2/1 -> delayMatch2/1
  Selector5/1 -> delayMatch3/1
  Selector4/1 -> delayMatch4/1
  t6/1 -> delayMatch5/1
  delayMatch/1 -> delayMatch6/1
  delayMatch1/1 -> delayMatch7/1
  delayMatch2/1 -> delayMatch8/1
  delayMatch3/1 -> delayMatch9/1
  delayMatch4/1 -> delayMatch10/1
  delayMatch5/1 -> delayMatch11/1
  delayMatch6/1 -> delayMatch12/1
  delayMatch7/1 -> delayMatch13/1
  delayMatch8/1 -> delayMatch14/1
  delayMatch9/1 -> delayMatch15/1
  delayMatch10/1 -> delayMatch16/1
  delayMatch11/1 -> delayMatch17/1
  theta_el_with_offset/1 -> cos_to_sincos/1(In1)
  u_dc_link_voltage/1 -> t6/4, t6/3, t6/2, t6/1
  Index/1 -> adder/1

== system gm_Phase_voltages_per_switching_state_MPC_6Phase/HDL_DUT/Detect Rise Positive1/Positive ==
  u : Inport  OutDataTypeStr=boolean  SampleTime=1e-08
  Compare : RelationalOperator  Operator=>  OutDataTypeStr=boolean  ZeroCross=off
  Constant : Constant  DisableCoverage=on  Value=0  OutDataTypeStr=Inherit: Inherit via back propagation  SampleTime=-1  PreserveConstantTs=on
  y : Outport  SampleTime=1e-08
  wires:
  Compare/1 -> y/1
  Constant/1 -> Compare/2
  u/1 -> Compare/1

== system gm_Phase_voltages_per_switching_state_MPC_6Phase/HDL_DUT/Detect Rise Positive2/Positive ==
  u : Inport  OutDataTypeStr=boolean  SampleTime=1e-08
  Compare : RelationalOperator  Operator=>  OutDataTypeStr=boolean  ZeroCross=off
  Constant : Constant  DisableCoverage=on  Value=0  OutDataTypeStr=Inherit: Inherit via back propagation  SampleTime=-1  PreserveConstantTs=on
  y : Outport  SampleTime=1e-08
  wires:
  Compare/1 -> y/1
  Constant/1 -> Compare/2
  u/1 -> Compare/1

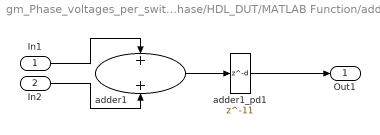
== system gm_Phase_voltages_per_switching_state_MPC_6Phase/HDL_DUT/MATLAB Function/adder1 ==
  In1 : Inport
  In2 : Inport  Port=2
  adder1 : Sum  OutDataTypeStr=single  SampleTime=1e-08
  adder1_pd1 : Delay  DelayLength=11
  Out1 : Outport
  wires:
  In1/1 -> adder1/1
  In2/1 -> adder1/2
  adder1/1 -> adder1_pd1/1
  adder1_pd1/1 -> Out1/1

== system gm_Phase_voltages_per_switching_state_MPC_6Phase/HDL_DUT/MATLAB Function/adder2 ==
  In1 : Inport
  In2 : Inport  Port=2
  adder2 : Sum  OutDataTypeStr=single  SampleTime=1e-08
  adder2_pd1 : Delay  DelayLength=11
  Out1 : Outport
  wires:
  In1/1 -> adder2/1
  In2/1 -> adder2/2
  adder2/1 -> adder2_pd1/1
  adder2_pd1/1 -> Out1/1

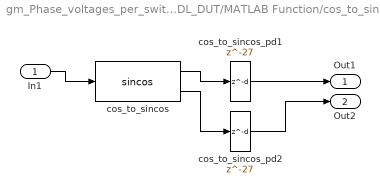
== system gm_Phase_voltages_per_switching_state_MPC_6Phase/HDL_DUT/MATLAB Function/cos_to_sincos ==
  In1 : Inport
  cos_to_sincos : Trigonometry  Operator=sincos  SampleTime=1e-08
  cos_to_sincos_pd1 : Delay  DelayLength=27
  cos_to_sincos_pd2 : Delay  DelayLength=27
  Out1 : Outport
  Out2 : Outport  Port=2
  wires:
  In1/1 -> cos_to_sincos/1
  cos_to_sincos/1 -> cos_to_sincos_pd1/1
  cos_to_sincos_pd1/1 -> Out1/1
  cos_to_sincos/2 -> cos_to_sincos_pd2/1
  cos_to_sincos_pd2/1 -> Out2/1

== system gm_Phase_voltages_per_switching_state_MPC_6Phase/HDL_DUT/MATLAB Function/multiplier ==
  In1 : Inport
  In2 : Inport  Port=2
  multiplier : Product  Inputs=**  OutDataTypeStr=single  SampleTime=1e-08
  multiplier_pd1 : Delay  DelayLength=8
  Out1 : Outport
  wires:
  In1/1 -> multiplier/1
  In2/1 -> multiplier/2
  multiplier/1 -> multiplier_pd1/1
  multiplier_pd1/1 -> Out1/1

== system gm_Phase_voltages_per_switching_state_MPC_6Phase/HDL_DUT/MATLAB Function/multiplier1 ==
  In1 : Inport
  In2 : Inport  Port=2
  multiplier1 : Product  Inputs=**  OutDataTypeStr=single  SampleTime=1e-08
  multiplier1_pd1 : Delay  DelayLength=8
  Out1 : Outport
  wires:
  In1/1 -> multiplier1/1
  In2/1 -> multiplier1/2
  multiplier1/1 -> multiplier1_pd1/1
  multiplier1_pd1/1 -> Out1/1

== system gm_Phase_voltages_per_switching_state_MPC_6Phase/HDL_DUT/MATLAB Function/multiplier2 ==
  In1 : Inport
  In2 : Inport  Port=2
  multiplier2 : Product  Inputs=**  OutDataTypeStr=single  SampleTime=1e-08
  multiplier2_pd1 : Delay  DelayLength=8
  Out1 : Outport
  wires:
  In1/1 -> multiplier2/1
  In2/1 -> multiplier2/2
  multiplier2/1 -> multiplier2_pd1/1
  multiplier2_pd1/1 -> Out1/1

== system gm_Phase_voltages_per_switching_state_MPC_6Phase/HDL_DUT/MATLAB Function/multiplier3 ==
  In1 : Inport
  In2 : Inport  Port=2
  multiplier3 : Product  Inputs=**  OutDataTypeStr=single  SampleTime=1e-08
  multiplier3_pd1 : Delay  DelayLength=8
  Out1 : Outport
  wires:
  In1/1 -> multiplier3/1
  In2/1 -> multiplier3/2
  multiplier3/1 -> multiplier3_pd1/1
  multiplier3_pd1/1 -> Out1/1

== system gm_Phase_voltages_per_switching_state_MPC_6Phase/HDL_DUT/MATLAB Function/multiplier4 ==
  In1 : Inport
  In2 : Inport  Port=2
  multiplier4 : Product  Inputs=**  OutDataTypeStr=single  SampleTime=1e-08
  multiplier4_pd1 : Delay  DelayLength=8
  Out1 : Outport
  wires:
  In1/1 -> multiplier4/1
  In2/1 -> multiplier4/2
  multiplier4/1 -> multiplier4_pd1/1
  multiplier4_pd1/1 -> Out1/1

== system gm_Phase_voltages_per_switching_state_MPC_6Phase/HDL_DUT/MATLAB Function/uminus ==
  In1 : Inport
  uminus : UnaryMinus  SampleTime=1e-08
  Out1 : Outport
  wires:
  In1/1 -> uminus/1
  uminus/1 -> Out1/1
